simulink model "V8_mdl"  (R2026a)
settings: Solver=FixedStepAuto  StartTime=0  StopTime=68.07  FixedStep=0.1
undefined symbols (not defined in the file): DiscIntNeverNeededParam, engineInertia, frontWheelMass, quarterCarMass, RAD2DEG_V, RAD2RPM, transmissionRatio, vehicle, vehicleMass, wheelRadius
settings Model: Creator=lholliday  LastModifiedBy=lholliday
settings SolverCC: ZeroCrossAlgorithm=Adaptive
settings DebuggingCC: IgnoredZcDiagnostic=none

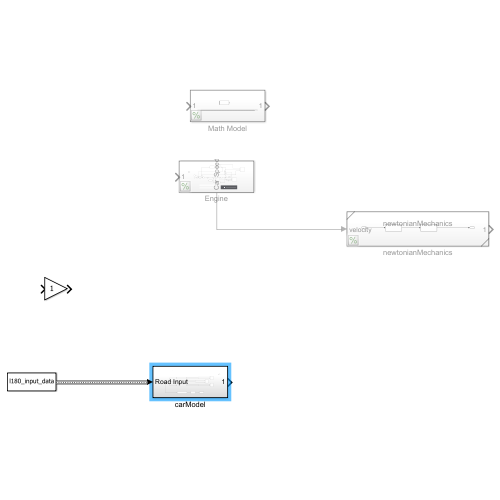
[thumbnail: Simulink's stored preview of the top-level diagram]
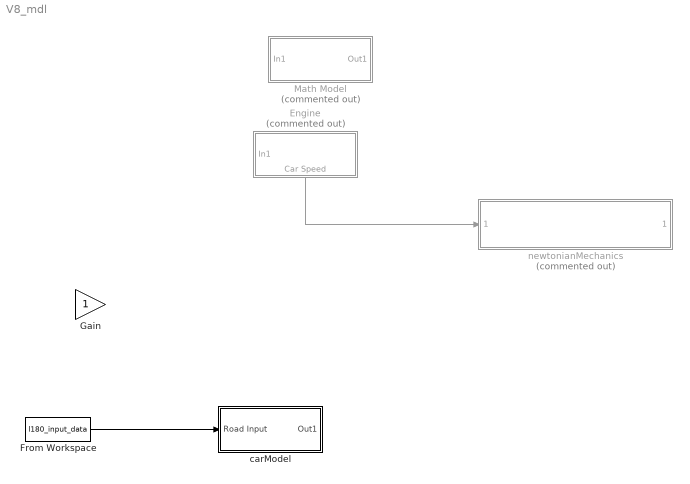
== system V8_mdl ==
  Engine : Subsystem  Commented=on
      settings: PortSchema="{\"entries\":[{\"content\":{\"sides\":[{\"content\":{\"connectorIds\":[\"In1\"]},\"type\":\"ConnectorPlacement.EquallySpacedRectSide\",\"uuid\":\"cadefebd-ad35-45dd-ae6a-9cccba43091e\"},{\"content\":{\"side\":\"RIGHT\"},\"type\":\"ConnectorPlacement.EquallySpacedRectSide\",\"uuid\":\"19d80bd4-267d-442e-b097-df40bf687d47\"},{\"content\":{\"side\":\"TOP\"},\"type\":\"ConnectorPlacement.EquallySpacedRectSide\",\"uuid\":\"6fb819b3-fb92-45d9-900f-1a7e7377e005\"},{\"content\":{\"connectorIds\":[\"Out1\"],\"side\":\"BOTTOM\"},\"type\":\"ConnectorPlacement.EquallySpacedRectSide\",\"uuid\":\"7f1958ad-d9a3-4585-8001-e48a895689d5\"}]},\"type\":\"ConnectorPlacement.EquallySpacedConnector\",\"uuid\":\"841cb558-8111-43be-8d99-0da8351c5108\"}],\"packageUris\":[\"http://schema.mathworks.com/mf0/Connector/R2020b\"],\"version\":\"1.0\"}"
  From Workspace : FromWorkspace  VariableName=l180_input_data  OutDataTypeStr=Bus: l180_bus
  Gain : Gain
  Math Model : Subsystem  Commented=on
  carModel : Subsystem
  newtonianMechanics : Subsystem  Commented=on  ReferencedSubsystem=newtonianMechanics
  wires:
  Engine/1(Car Speed) -> newtonianMechanics/1
  From Workspace/1 -> carModel/1(Road Input)

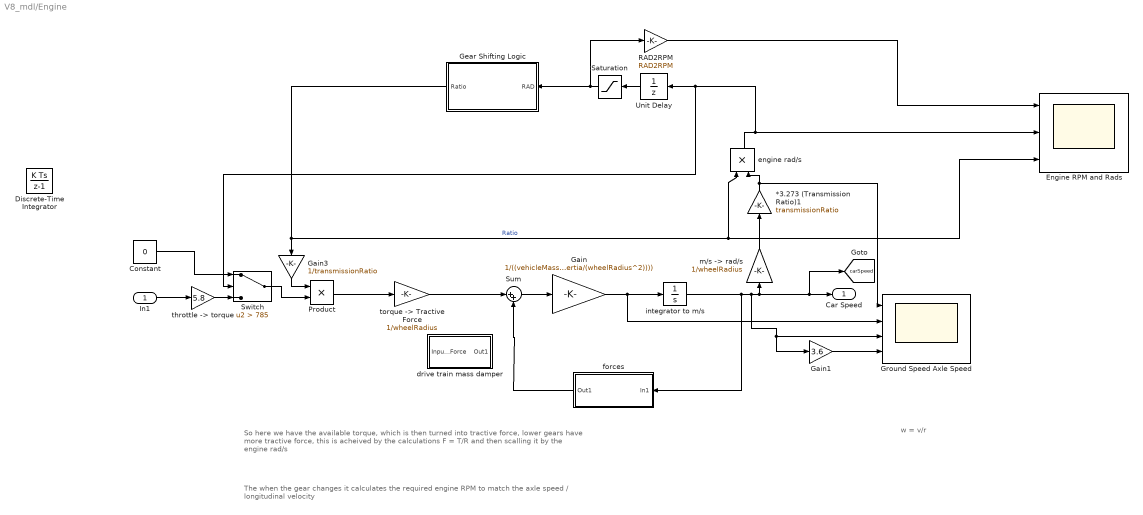
== system V8_mdl/Engine ==
  note: w = v/r
  note: The when the gear changes it calculates the required engine RPM to match the axle speed / longitudinal velocity
  note: So here we have the available torque, which is then turned into tractive force, lower gears have more tractive force, this is acheived by the calculations F = T/R and then scalling it by the engine rad/s
  In1 : Inport
  *3.273 (Transmission Ratio)1 : Gain  Gain=transmissionRatio
  Constant : Constant  Value=0
  Discrete-Time Integrator : DiscreteIntegrator  InitialConditionSource=external  SampleTime=-1  ICPrevOutput=DiscIntNeverNeededParam  ICPrevScaledInput=DiscIntNeverNeededParam
  Engine RPM and Rads : Scope  NumInputPorts=3
      settings: ActiveDisplayYMinimum=5459.4365717640658  ActiveDisplayYMaximum=8132.1776448532992
  Gain : Gain  Gain=1/((vehicleMass + (engineInertia/(wheelRadius^2))))
  Gain1 : Gain  Gain=3.6
  Gain3 : Gain  Gain=1/transmissionRatio
  Gear Shifting Logic : Subsystem
  Ground Speed Axle Speed : Scope  NumInputPorts=4
      settings: ActiveDisplayYMinimum=-98.141798139810533  ActiveDisplayYMaximum=883.27618325829508  DataLoggingVariableName=ScopeData5
  Product : Product
  RAD2RPM : Gain  Gain=RAD2RPM
  Saturation : Saturate  UpperLimit=7600  LowerLimit=0
  Sum : Sum  Inputs=|++
  Switch : Switch  Criteria=u2 > Threshold  Threshold=785  SaturateOnIntegerOverflow=off  InputSameDT=off
  Unit Delay : UnitDelay  SampleTime=-1
  drive train mass damper : Subsystem
  engine rad/s : Product
  forces : Subsystem
  integrator to m/s : Integrator
  "m/s -> rad/s" : Gain  Gain=1/wheelRadius
  "throttle -> torque" : Gain  Gain=5.8
  "torque -> Tractive Force" : Gain  Gain=1/wheelRadius
  Car Speed : Outport
  tag scope: carSpeed=global
  wires:
  In1/1 -> "throttle -> torque"/1
  Gain/1 -> Ground Speed Axle Speed/2, integrator to m/s/1
  forces/1(Out1) -> Sum/2
  Gear Shifting Logic/1(Ratio) -> Engine RPM and Rads/3, engine rad/s/1, Gain3/1  "Ratio"
  integrator to m/s/1 -> forces/1(In1), Gain1/1, Ground Speed Axle Speed/3, [carSpeed], Car Speed/1, "m/s -> rad/s"/1
  "m/s -> rad/s"/1 -> *3.273 (Transmission Ratio)1/1
  Unit Delay/1 -> Saturation/1
  Saturation/1 -> RAD2RPM/1, Gear Shifting Logic/1(RAD)
  Gain1/1 -> Ground Speed Axle Speed/4
  Product/1 -> "torque -> Tractive Force"/1
  engine rad/s/1 -> Switch/2, Unit Delay/1, Engine RPM and Rads/2
  RAD2RPM/1 -> Engine RPM and Rads/1
  *3.273 (Transmission Ratio)1/1 -> engine rad/s/2, Ground Speed Axle Speed/1
  Gain3/1 -> Product/1
  Sum/1 -> Gain/1
  Switch/1 -> Product/2
  "throttle -> torque"/1 -> Switch/3
  Constant/1 -> Switch/1
  "torque -> Tractive Force"/1 -> Sum/1

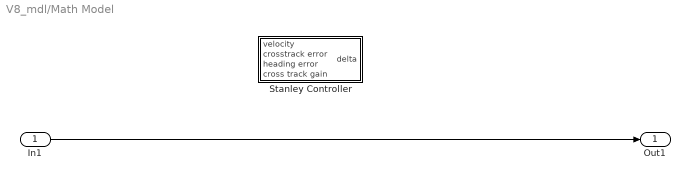
== system V8_mdl/Math Model ==
  In1 : Inport
  Stanley Controller : Subsystem
  Out1 : Outport
  wires:
  In1/1 -> Out1/1

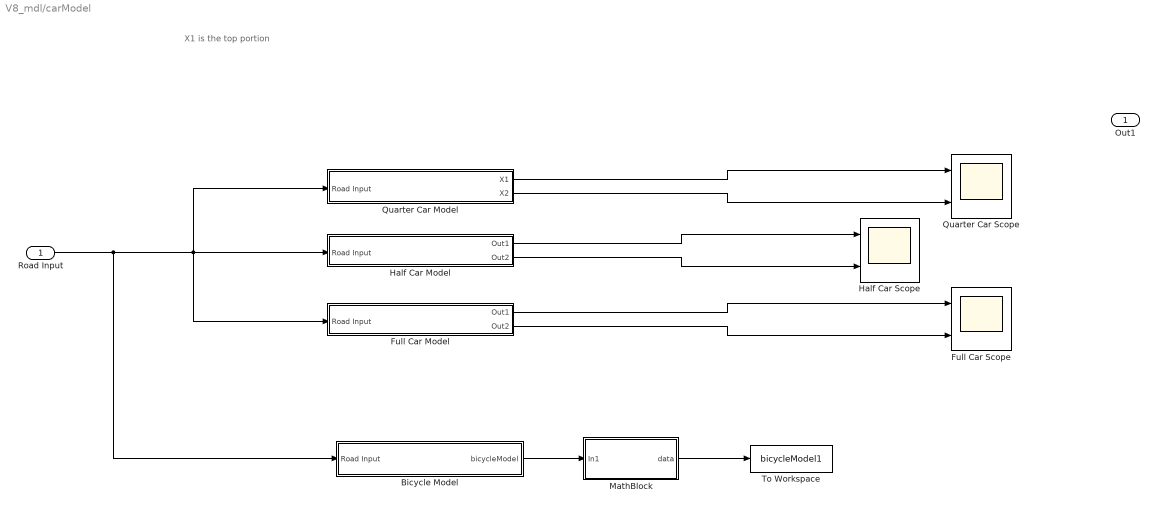
== system V8_mdl/carModel ==
  note: X1 is the top portion
  Road Input : Inport
  Bicycle Model : Subsystem
  Full Car Model : Subsystem
  Full Car Scope : Scope  NumInputPorts=2
      settings: ActiveDisplayYMinimum=-0.21783096010722808  ActiveDisplayYMaximum=1.9604786409650532  DataLoggingVariableName=ScopeData8
  Half Car Model : Subsystem
  Half Car Scope : Scope  NumInputPorts=2
      settings: ActiveDisplayYMinimum=-0.21783096010722808  ActiveDisplayYMaximum=1.9604786409650532  DataLoggingVariableName=ScopeData7
  MathBlock : Subsystem
  Quarter Car Model : Subsystem
  Quarter Car Scope : Scope  NumInputPorts=2
      settings: ActiveDisplayYMinimum=-0.21783096010722808  ActiveDisplayYMaximum=1.9604786409650532  DataLoggingVariableName=ScopeData6
  To Workspace : ToWorkspace  VariableName=bicycleModel1  SaveFormat=Timeseries  SampleTime=-1
  Out1 : Outport
  wires:
  Quarter Car Model/1(X1) -> Quarter Car Scope/1
  Quarter Car Model/2(X2) -> Quarter Car Scope/2
  Road Input/1 -> Bicycle Model/1(Road Input), Full Car Model/1(Road Input), Half Car Model/1(Road Input), Quarter Car Model/1(Road Input)
  Half Car Model/1(Out1) -> Half Car Scope/1
  Half Car Model/2(Out2) -> Half Car Scope/2
  Full Car Model/2(Out2) -> Full Car Scope/2
  Full Car Model/1(Out1) -> Full Car Scope/1
  Bicycle Model/1(bicycleModel) -> MathBlock/1(In1)
  MathBlock/1(data) -> To Workspace/1

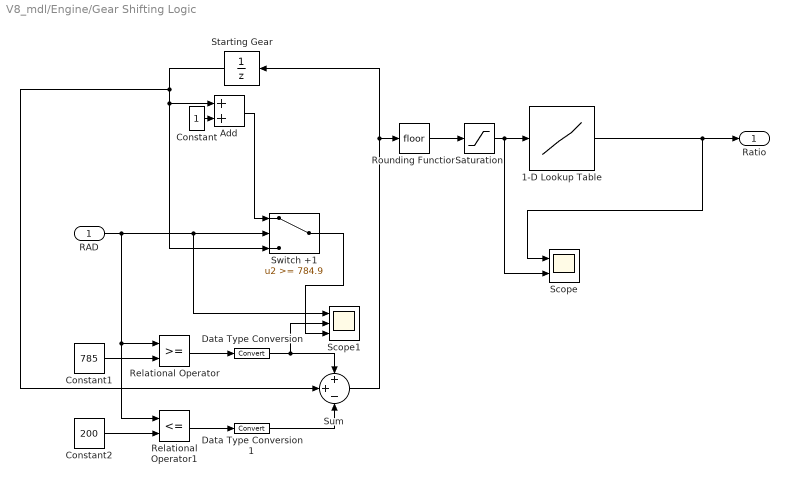
== system V8_mdl/Engine/Gear Shifting Logic ==
  RAD : Inport
  1-D Lookup Table : Lookup_n-D  NumberOfTableDimensions=1  BreakpointsForDimension1=[1;2;3;4;5;6]  Table=[2.5750000000000002;1.99;1.597;1.3300000000000001;1.143;1]  InternalRulePriority=Speed  RndMeth=Simplest
  Add : Sum
  Constant : Constant
  Constant1 : Constant  Value=785
  Constant2 : Constant  Value=200
  Data Type Conversion : DataTypeConversion  SaturateOnIntegerOverflow=off  RndMeth=Floor
  Data Type Conversion1 : DataTypeConversion  SaturateOnIntegerOverflow=off  RndMeth=Floor
  Relational Operator : RelationalOperator  OutDataTypeStr=fixdt(1,16)  RndMeth=Simplest  InputSameDT=off
  Relational Operator1 : RelationalOperator  Operator=<=  OutDataTypeStr=boolean  RndMeth=Simplest  InputSameDT=off
  Rounding Function : Rounding
  Saturation : Saturate  UpperLimit=6  LowerLimit=1
  Scope : Scope  NumInputPorts=2
      settings: ActiveDisplayYMinimum=0.80312500000000009  ActiveDisplayYMaximum=2.771875
  Scope1 : Scope  NumInputPorts=3
      settings: ActiveDisplayYMinimum=-98.326682289767959  ActiveDisplayYMaximum=884.94014060791187  DataLoggingVariableName=ScopeData3
  Starting Gear : UnitDelay  InitialCondition=1  SampleTime=-1
  Sum : Sum  Inputs=++-
  "Switch +1 " : Switch  Threshold=784.9  ZeroCross=off  SaturateOnIntegerOverflow=off  InputSameDT=off
  Ratio : Outport
  wires:
  Constant/1 -> Add/2
  Starting Gear/1 -> "Switch +1 "/3, Add/1, Sum/2
  "Switch +1 "/1 -> Scope1/3
  Saturation/1 -> Scope/2, 1-D Lookup Table/1
  Rounding Function/1 -> Saturation/1
  Add/1 -> "Switch +1 "/1
  1-D Lookup Table/1 -> Scope/1, Ratio/1
  Constant1/1 -> Relational Operator/2
  RAD/1 -> Relational Operator1/1, Relational Operator/1, "Switch +1 "/2, Scope1/1
  Constant2/1 -> Relational Operator1/2
  Relational Operator1/1 -> Data Type Conversion1/1
  Sum/1 -> Rounding Function/1, Starting Gear/1
  Relational Operator/1 -> Data Type Conversion/1
  Data Type Conversion/1 -> Scope1/2, Sum/1
  Data Type Conversion1/1 -> Sum/3

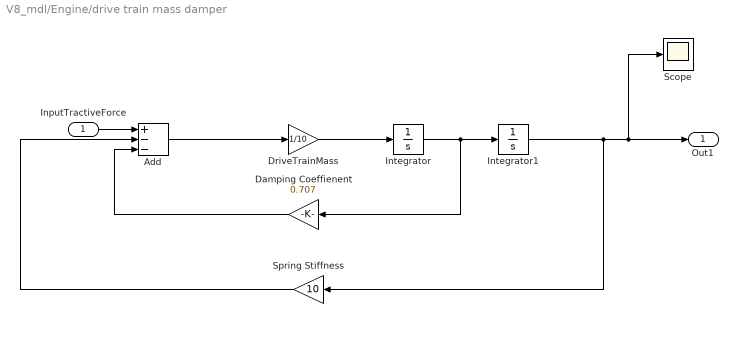
== system V8_mdl/Engine/drive train mass damper ==
  InputTractiveForce : Inport
  Add : Sum  Inputs=+--
  Damping Coeffienent : Gain  Gain=0.707
  DriveTrainMass : Gain  Gain=1/10
  Integrator : Integrator
  Integrator1 : Integrator
  Scope : Scope
      settings: ActiveDisplayYMinimum=-1  ActiveDisplayYMaximum=1  DataLoggingVariableName=ScopeData4
  Spring Stiffness : Gain  Gain=10
  Out1 : Outport
  wires:
  InputTractiveForce/1 -> Add/1
  Add/1 -> DriveTrainMass/1
  DriveTrainMass/1 -> Integrator/1
  Integrator/1 -> Damping Coeffienent/1, Integrator1/1
  Damping Coeffienent/1 -> Add/3
  Spring Stiffness/1 -> Add/2
  Integrator1/1 -> Spring Stiffness/1, Scope/1, Out1/1

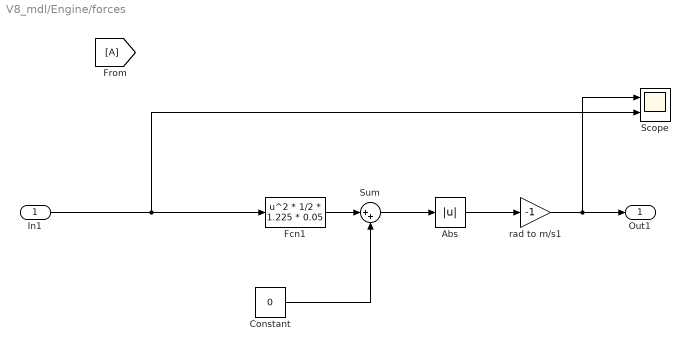
== system V8_mdl/Engine/forces ==
  In1 : Inport
  Abs : Abs  SaturateOnIntegerOverflow=off
  Constant : Constant  Value=0
  Fcn1 : Fcn  Expr=u^2 * 1/2 * 1.225 * 0.05
  From : From
  Scope : Scope  NumInputPorts=2
      settings: ActiveDisplayYMinimum=-59.044453764161155  ActiveDisplayYMaximum=6.5604948626845712  DataLoggingVariableName=ScopeData2
  Sum : Sum  Inputs=|++
  rad to m/s1 : Gain  Gain=-1
  Out1 : Outport
  wires:
  In1/1 -> Fcn1/1, Scope/2
  Abs/1 -> rad to m/s1/1
  Fcn1/1 -> Sum/1
  Sum/1 -> Abs/1
  rad to m/s1/1 -> Scope/1, Out1/1
  Constant/1 -> Sum/2

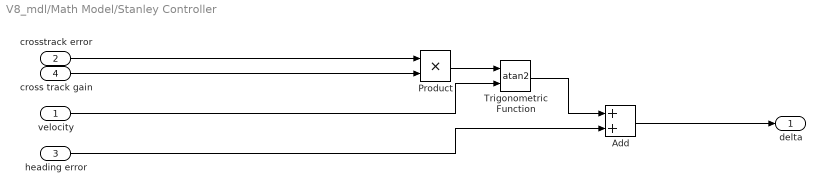
== system V8_mdl/Math Model/Stanley Controller ==
  velocity : Inport
  crosstrack error : Inport  Port=2
  heading error : Inport  Port=3
  cross track gain : Inport  Port=4
  Add : Sum
  Product : Product
  Trigonometric Function : Trigonometry  Operator=atan2
  delta : Outport
  wires:
  crosstrack error/1 -> Product/1
  cross track gain/1 -> Product/2
  Product/1 -> Trigonometric Function/1
  heading error/1 -> Add/2
  velocity/1 -> Trigonometric Function/2
  Add/1 -> delta/1
  Trigonometric Function/1 -> Add/1

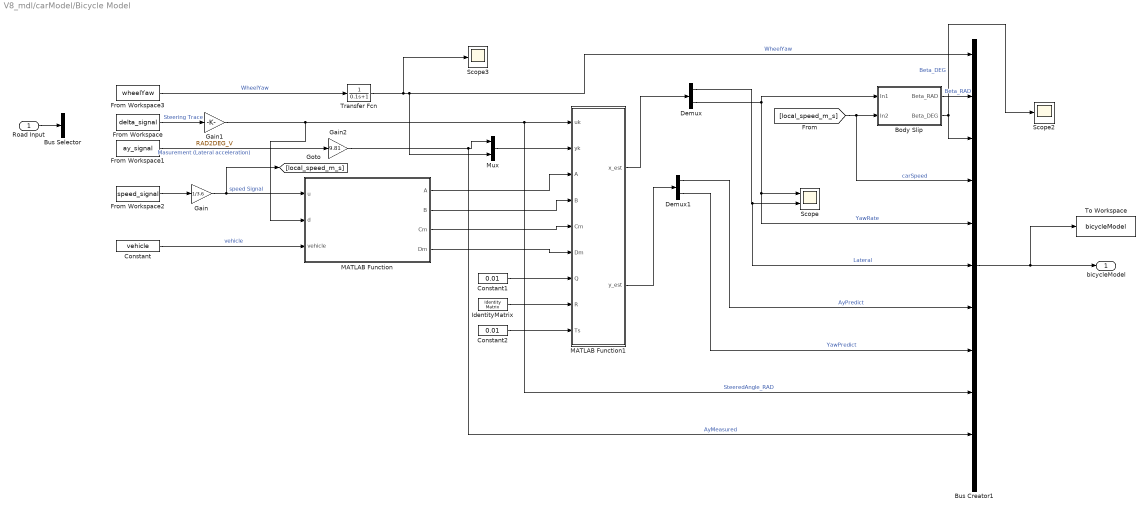
== system V8_mdl/carModel/Bicycle Model ==
  Road Input : Inport
  Body Slip : Subsystem
  Bus Creator1 : BusCreator  Inputs=11
  Bus Selector : BusSelector  OutputSignals=Ground_Speed,Steering_Angle
  Constant : Constant  Value=vehicle  OutDataTypeStr=Bus: vehicleBus
  Constant1 : Constant  Value=0.01
  Constant2 : Constant  Value=0.01
  Demux : Demux  Outputs=2
  Demux1 : Demux  Outputs=2
  From Workspace : FromWorkspace  VariableName=delta_signal  SampleTime=-1
  From Workspace1 : FromWorkspace  VariableName=ay_signal  SampleTime=-1
  From Workspace2 : FromWorkspace  VariableName=speed_signal  SampleTime=-1
  From Workspace3 : FromWorkspace  VariableName=wheelYaw  SampleTime=-1
  Gain : Gain  Gain=1/3.6
  Gain1 : Gain  Gain=RAD2DEG_V
  Gain2 : Gain  Gain=9.81
  IdentityMatrix : IdentityMatrix  OutputDimensions=2
  MATLAB Function : MATLAB Function  TreatAsAtomicUnit=on
  MATLAB Function1 : MATLAB Function  TreatAsAtomicUnit=on
  Mux : Mux  Inputs=2
  Scope : Scope  NumInputPorts=2
      settings: ActiveDisplayYMinimum=-3.7432847245504721  ActiveDisplayYMaximum=2.7904018957839103  DataLoggingVariableName=ScopeData10
  Scope2 : Scope
      settings: ActiveDisplayYMinimum=-11.185998106528842  ActiveDisplayYMaximum=6.4154629689210907  DataLoggingVariableName=ScopeData12
  Scope3 : Scope
      settings: ActiveDisplayYMinimum=-1  ActiveDisplayYMaximum=1  DataLoggingVariableName=ScopeData13
  To Workspace : ToWorkspace  VariableName=bicycleModel  SaveFormat=Timeseries  SampleTime=-1
  Transfer Fcn : TransferFcn  Denominator=[0.1 1]
  bicycleModel : Outport
  wires:
  From Workspace2/1 -> Gain/1
  From Workspace/1 -> Gain1/1  "Steering Trace"
  MATLAB Function1/1(x_est) -> Demux/1
  Gain2/1 -> Mux/1, Bus Creator1/10  "AyMeasured"
  MATLAB Function/3(Cm) -> MATLAB Function1/5(Cm)
  Constant/1 -> MATLAB Function/3(vehicle)  "vehicle"
  Demux/1 -> Bus Creator1/6, Scope/2  "Lateral"
  Demux/2 -> Body Slip/1(In1), Bus Creator1/5, Scope/1  "YawRate"
  Bus Creator1/1 -> To Workspace/1, bicycleModel/1
  Body Slip/1(Beta_RAD) -> Bus Creator1/2  "Beta_RAD"
  [local_speed_m_s] -> Bus Creator1/4, Body Slip/2(In2)  "carSpeed"
  Body Slip/2(Beta_DEG) -> Scope2/1, Bus Creator1/3  "Beta_DEG"
  MATLAB Function/1(A) -> MATLAB Function1/3(A)
  MATLAB Function/2(B) -> MATLAB Function1/4(B)
  Gain1/1 -> MATLAB Function/2(d), MATLAB Function1/1(uk), Bus Creator1/9  "SteeredAngle_RAD"
  Gain/1 -> MATLAB Function/1(u), [local_speed_m_s]  "speed Signal"
  From Workspace1/1 -> Gain2/1  "Masurement (Lateral acceleration)"
  From Workspace3/1 -> Transfer Fcn/1  "WheelYaw"
  Mux/1 -> MATLAB Function1/2(yk)
  Transfer Fcn/1 -> Scope3/1, Mux/2, Bus Creator1/1  "WheelYaw"
  MATLAB Function1/2(y_est) -> Demux1/1
  Demux1/1 -> Bus Creator1/7  "AyPredict"
  Demux1/2 -> Bus Creator1/8  "YawPredict"
  MATLAB Function/4(Dm) -> MATLAB Function1/6(Dm)
  ? -> Bus Creator1/11
  Constant1/1 -> MATLAB Function1/7(Q)
  IdentityMatrix/1 -> MATLAB Function1/8(R)
  Constant2/1 -> MATLAB Function1/9(Ts)
  Road Input/1 -> Bus Selector/1

== system V8_mdl/carModel/Full Car Model ==
  Road Input : Inport
  Out1 : Outport
  Out2 : Outport  Port=2
  wires:
  Road Input/1 -> Out1/1

== system V8_mdl/carModel/Half Car Model ==
  Road Input : Inport
  Out1 : Outport
  Out2 : Outport  Port=2
  wires:
  Road Input/1 -> Out1/1

== system V8_mdl/carModel/MathBlock ==
  In1 : Inport
  Tyres : Subsystem
  data : Outport
  wires:
  In1/1 -> Tyres/1(In1)
  Tyres/1(Out1) -> data/1

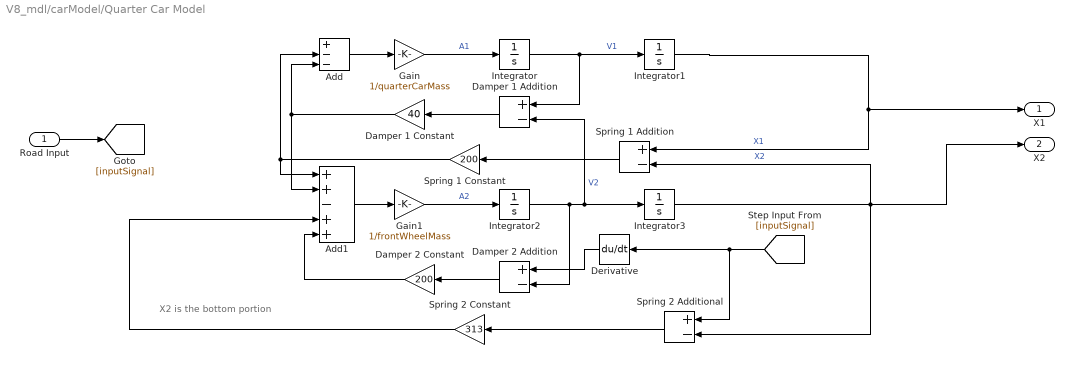
== system V8_mdl/carModel/Quarter Car Model ==
  note: X2 is the bottom portion
  Road Input : Inport
  Add : Sum  Inputs=+--
  Add1 : Sum  Inputs=++-++
  Damper 1 Addition : Sum  Inputs=+-
  Damper 1 Constant : Gain  Gain=40
  Damper 2 Addition : Sum  Inputs=+-
  Damper 2 Constant : Gain  Gain=200
  Derivative : Derivative
  Gain : Gain  Gain=1/quarterCarMass
  Gain1 : Gain  Gain=1/frontWheelMass
  Integrator{,1..3} (4 alike) : Integrator
  Spring 1 Addition : Sum  Inputs=+-
  Spring 1 Constant : Gain  Gain=200
  Spring 2 Additional : Sum  Inputs=+-
  Spring 2 Constant : Gain  Gain=313
  X1 : Outport
  X2 : Outport  Port=2
  wires:
  Derivative/1 -> Damper 2 Addition/1
  Add/1 -> Gain/1
  Damper 2 Constant/1 -> Add1/5
  Add1/1 -> Gain1/1
  Damper 1 Constant/1 -> Add/3, Add1/2
  Spring 2 Additional/1 -> Spring 2 Constant/1
  [inputSignal] -> Spring 2 Additional/1, Derivative/1
  Integrator3/1 -> X2/1, Spring 2 Additional/2, Spring 1 Addition/2  "X2"
  Damper 2 Addition/1 -> Damper 2 Constant/1
  Spring 2 Constant/1 -> Add1/4
  Gain/1 -> Integrator/1  "A1"
  Integrator1/1 -> X1/1, Spring 1 Addition/1  "X1"
  Gain1/1 -> Integrator2/1  "A2"
  Integrator2/1 -> Damper 2 Addition/2, Damper 1 Addition/2, Integrator3/1  "V2"
  Integrator/1 -> Damper 1 Addition/1, Integrator1/1  "V1"
  Damper 1 Addition/1 -> Damper 1 Constant/1
  Spring 1 Constant/1 -> Add/2, Add1/1
  Spring 1 Addition/1 -> Spring 1 Constant/1
  Road Input/1 -> [inputSignal]

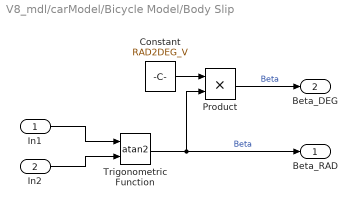
== system V8_mdl/carModel/Bicycle Model/Body Slip ==
  In1 : Inport
  In2 : Inport  Port=2
  Constant : Constant  Value=RAD2DEG_V
  Product : Product
  Trigonometric Function : Trigonometry  Operator=atan2
  Beta_RAD : Outport
  Beta_DEG : Outport  Port=2
  wires:
  Trigonometric Function/1 -> Product/2, Beta_RAD/1  "Beta"
  In1/1 -> Trigonometric Function/1
  In2/1 -> Trigonometric Function/2
  Constant/1 -> Product/1
  Product/1 -> Beta_DEG/1  "Beta"

== system V8_mdl/carModel/MathBlock/Tyres ==
  In1 : Inport
  Tyre Slip Angles : Subsystem
  Out1 : Outport
  wires:
  In1/1 -> Tyre Slip Angles/1(In1)
  Tyre Slip Angles/1(tyres) -> Out1/1

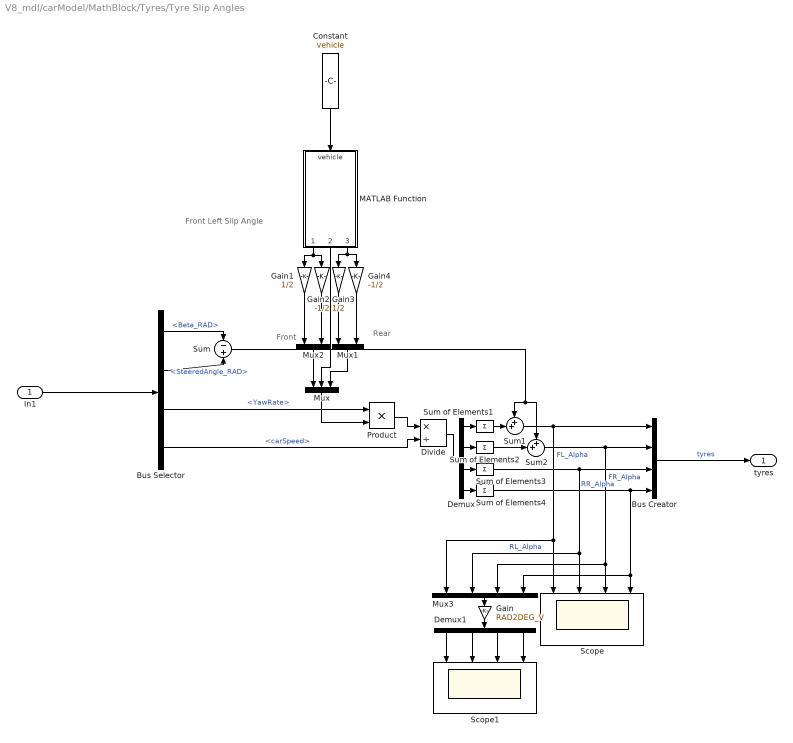
== system V8_mdl/carModel/MathBlock/Tyres/Tyre Slip Angles ==
  note: Rear
  note: Front Left Slip Angle
  note: Front
  In1 : Inport
  Bus Creator : BusCreator  Inputs=4
  Bus Selector : BusSelector  OutputSignals=Beta_RAD,SteeredAngle_RAD,YawRate,carSpeed
  Constant : Constant  Value=vehicle  OutDataTypeStr=Bus: vehicleBus
  Demux : Demux
  Demux1 : Demux
  Divide : Product  Inputs=*/
  Gain : Gain  Gain=RAD2DEG_V
  Gain1 : Gain  Gain=1/2
  Gain2 : Gain  Gain=-1/2
  Gain3 : Gain  Gain=1/2
  Gain4 : Gain  Gain=-1/2
  MATLAB Function : MATLAB Function  TreatAsAtomicUnit=on
  Mux : Mux  Inputs=3
  Mux1 : Mux  Inputs=2
      settings: DisplayOption=signals
  Mux2 : Mux  Inputs=2
      settings: DisplayOption=signals
  Mux3 : Mux
  Product : Product
  Scope : Scope  NumInputPorts=4
      settings: ActiveDisplayYMinimum=-0.38056926667022484  ActiveDisplayYMaximum=0.25240760580118693  DataLoggingVariableName=ScopeData11
  Scope1 : Scope  NumInputPorts=4
      settings: ActiveDisplayYMinimum=-5.9723403916960152  ActiveDisplayYMaximum=5.79548963009766  DataLoggingVariableName=ScopeData11
  Sum : Sum  Inputs=-|+
  Sum of Elements{1..4} (4 alike) : Sum  Inputs=+
  Sum1 : Sum  Inputs=++|
  Sum2 : Sum  Inputs=++|
  tyres : Outport
  wires:
  Sum of Elements1/1 -> Sum1/2
  MATLAB Function/2(frontArm) -> Mux/2
  Bus Creator/1 -> tyres/1  "tyres"
  In1/1 -> Bus Selector/1
  MATLAB Function/1(trackWidth) -> Gain1/1, Gain2/1
  Sum/1 -> Sum2/1, Sum1/1
  Demux1/3 -> Scope1/3
  Constant/1 -> MATLAB Function/1(vehicle)
  Demux1/1 -> Scope1/1
  Mux/1 -> Product/2
  Bus Selector/1 -> Sum/1  "<Beta_RAD>"
  Demux1/4 -> Scope1/4
  Bus Selector/4 -> Divide/2  "<carSpeed>"
  Sum of Elements2/1 -> Sum2/2
  Demux/4 -> Sum of Elements4/1
  Gain2/1 -> Mux2/2
  Bus Selector/3 -> Product/1  "<YawRate>"
  Sum of Elements4/1 -> Bus Creator/4, Mux3/4, Scope/4  "RR_Alpha"
  Mux1/1 -> Mux/3
  Mux2/1 -> Mux/1
  Product/1 -> Divide/1
  Gain1/1 -> Mux2/1
  Gain3/1 -> Mux1/1
  Bus Selector/2 -> Sum/2  "<SteeredAngle_RAD>"
  Divide/1 -> Demux/1
  Demux1/2 -> Scope1/2
  Sum of Elements3/1 -> Bus Creator/3, Mux3/2, Scope/2  "RL_Alpha"
  Demux/3 -> Sum of Elements3/1
  Sum1/1 -> Bus Creator/1, Mux3/1, Scope/1  "FL_Alpha"
  Sum2/1 -> Mux3/3, Scope/3, Bus Creator/2  "FR_Alpha"
  Mux3/1 -> Gain/1
  MATLAB Function/3(rearArm) -> Gain4/1, Gain3/1
  Demux/2 -> Sum of Elements2/1
  Gain/1 -> Demux1/1
  Demux/1 -> Sum of Elements1/1
  Gain4/1 -> Mux1/2

== matlab function V8_mdl/carModel/MathBlock/Tyres/Tyre Slip Angles/MATLAB Function ==
  data: vehicle input; trackWidth output; frontArm output; rearArm output
function [trackWidth, frontArm, rearArm] = getValue(vehicle)
    

trackWidth = vehicle.ford.kinematics.body.trackWidth/1000;
    frontArm = vehicle.E06DAR.bicycleModel.frontArm/1000;
    rearArm  = vehicle.E06DAR.bicycleModel.rearArm/1000;



end

== matlab function V8_mdl/carModel/Bicycle Model/MATLAB Function ==
  data: A output; B output; u input; d input; Cm output; Dm output; vehicle input
function [A, B, Cm, Dm] = bicycleModelStateSpaceMatrix(u, d, vehicle)
    
    % eventString = strcmp(event, event);
    m =  vehicle.E06DAR.bicycleModel.totalMass;
    mf = vehicle.E06DAR.bicycleModel.frontAxleMass;
    mr = vehicle.E06DAR.bicycleModel.rearAxleMass;
    lf = vehicle.E06DAR.bicycleModel.frontArm/1000;
    lr = vehicle.E06DAR.bicycleModel.rearArm/1000;

    Iz = mf*lf^2 + mr* lr^2;
    Caf = 150000;
    Car = 150000;

    A11 = -(2*Caf + 2*Car)/(m*u);
    A12 = -(u + (2*Caf*lf - 2*Car*lr)/(m*u));
    A21 =  (2*lf*Caf - 2*lr*Car)/(Iz*u);
    A22 = -(2*lf^2*Caf + 2*lr^2*Car)/(Iz*u);

    A = [A11, A12; A21, A22];
    B = [2*Caf/m; 2*Caf*lf/Iz] * d;

    % Kalman measurement matrix for ay
    Cm = [A11, (A12+u); 0 , 1];
    Dm = [2*Caf/m; 0];
end

== matlab function V8_mdl/carModel/Bicycle Model/MATLAB Function1 ==
  data: uk input; yk input; A input; x_est output; B input; Cm input; Dm input; Q input; R input; Ts input; y_est output
function [x_est, y_est] = discreteKalmanFilter(uk, yk, A, B, Cm, Dm, Q, R, Ts)
%#codegen
% Discrete-time Kalman filter for a MATLAB Function block in Simulink.
%
% Inputs:
%   A, B   - continuous-time state matrices from bicycleModelStateSpaceMatrix
%   Cm, Dm - measurement matrices (map states -> measured outputs, e.g. YawRate, AyMeasured)
%   uk     - current input vector (e.g. [delta; speed] or however u is defined)
%   yk     - current measurement vector (e.g. [YawRate; AyMeasured])
%   Q      - process noise covariance (n x n), tune this
%   R      - measurement noise covariance (m x m), tune this
%   Ts     - sample time (s) for discretization
%
% Outputs:
%   x_est  - updated (a posteriori) state estimate
%   y_est  - predicted measurement from x_est (Cm*x_est + Dm*uk)

n = size(A,1);      % number of states
m = size(Cm,1);     % number of measurements

% --- persistent filter state (initialized on first call) ---
persistent x P
if isempty(x)
    x = zeros(n,1);
end
if isempty(P)
    P = eye(n);      % initial covariance guess, tune if needed
end

% --- discretize continuous A,B (simple Euler; fine for small Ts) ---
Ad = eye(n) + A*Ts;
Bd = B*Ts;

% =========================================================
% TIME UPDATE (predict)
% =========================================================
x_pred = Ad*x + Bd*uk;
P_pred = Ad*P*Ad' + Q;

% =========================================================
% MEASUREMENT UPDATE (correct)
% =========================================================
y_pred = Cm*x_pred + Dm*uk;      % predicted measurement
innov   = yk - y_pred;           % innovation

S = Cm*P_pred*Cm' + R;           % innovation covariance
K = (P_pred*Cm') / S;            % Kalman gain (S is m x m, usually small -> cheap to invert)

x_upd = x_pred + K*innov;
P_upd = (eye(n) - K*Cm) * P_pred;

% --- store for next call ---
x = x_upd;
P = P_upd;

% --- outputs ---
x_est = x_upd;
y_est = Cm*x_upd + Dm*uk;

end
